simulink model "New_SPRO4"  (R2026a)
settings: Solver=FixedStepAuto  StopTime=8  RelTol=1e-6
libraries: simulink x1, slpidlib x1
settings OptimizationCC: UseDivisionForNetSlopeComputation=on  GainParamInheritBuiltInType=on  UseFloatMulNetSlope=on  InlineInvariantSignals=on  NoFixptDivByZeroProtection=on  EfficientFloat2IntCast=on  LifeSpan=1
settings RTWCC: SystemTargetFile=ert.tlc  GenerateReport=on  Toolchain=ESP32  LaunchReport=on  Description=Embedded Coder
settings CodeAppCC: CustomSymbolStrGlobalVar=rt$N$M  CustomSymbolStrType=$N$M  CustomSymbolStrFcn=$N$M$F  CustomSymbolStrMacro=$N$M
settings ERTTargetCC: ERTFilePackagingFormat=CompactWithDataFile  GenerateSampleERTMain=on  IncludeMdlTerminateFcn=off  CombineSignalStateStructs=on  SupportAbsoluteTime=off  SupportComplex=off  SupportContinuousTime=on

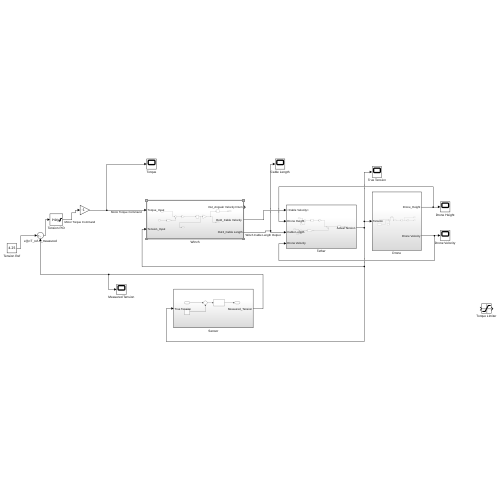
[thumbnail: Simulink's stored preview of the top-level diagram]
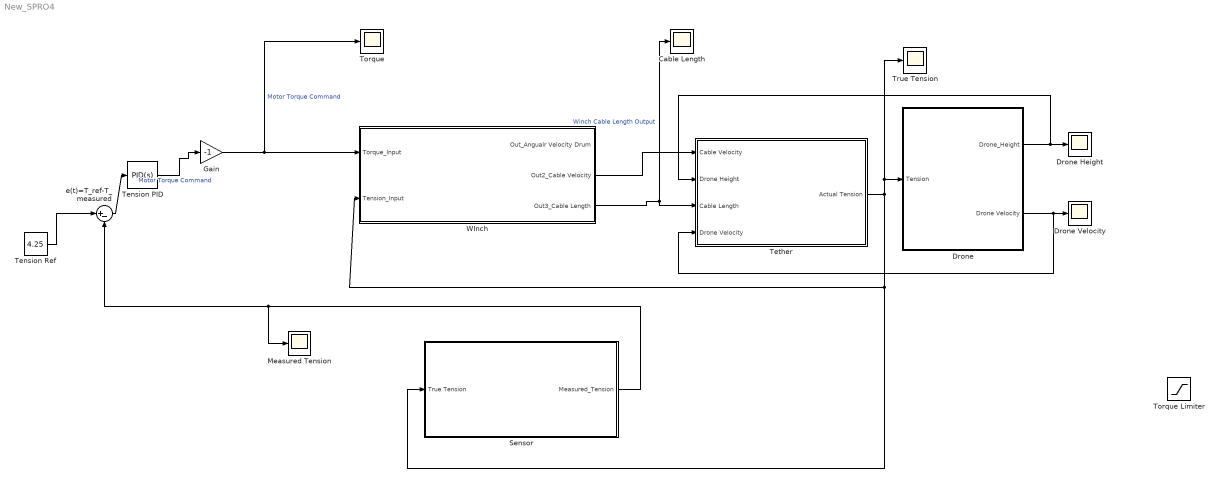
== system New_SPRO4 ==
  Cable Length : Scope
      settings: ActiveDisplayYMinimum=-13.075945732793034  ActiveDisplayYMaximum=11.241645498772957  DataLoggingVariableName=ScopeData5
  Drone : Subsystem
  Drone Height : Scope
      settings: ActiveDisplayYMinimum=-2.5970281910431563  ActiveDisplayYMaximum=9.2410311502356173  DataLoggingVariableName=ScopeData4
  Drone Velocity : Scope
      settings: ActiveDisplayYMinimum=-6.9644358509379627  ActiveDisplayYMaximum=6.4874715690258595  DataLoggingVariableName=ScopeData2
  Gain : Gain  Gain=-1
  Measured Tension : Scope
      settings: ActiveDisplayYMinimum=-21.256641439910606  ActiveDisplayYMaximum=16.681859235663254
  Sensor : Subsystem
  Tension PID : slpidlib/PID Controller  Controller=PID  Form=Parallel  TimeDomain=Continuous-time  UseExternalTs=off  SampleTime=-1  IntegratorMethod=Forward Euler  FilterMethod=Forward Euler  ControllerParametersSource=internal  P=0.005  I=0.002  UseKiTs=off  D=0.001  UseExternalDerivativeSource=off  N=10  UseFilter=on  TunerSelectOption=Transfer Function Based (PID Tuner App)  InitialConditionSource=internal  InitialConditionForIntegrator=0  InitialConditionForFilter=0  DifferentiatorICPrevScaledInput=0  ExternalReset=none  TrackingMode=off  Kt=1  LimitOutput=on  SatLimitsSource=internal  UpperSaturationLimit=0.0084  LowerSaturationLimit=-0.0084  LinearizeAsGain=on  AntiWindupMode=clamping  Kb=1  LimitIntegrator=on  UpperIntegratorSaturationLimit=0.0078  LowerIntegratorSaturationLimit=-0.0078  POutMin=[]  POutMax=[]  IOutMin=[]  IOutMax=[]  DOutMin=[]  DOutMax=[]  NOutMin=[]  NOutMax=[]  SumOutMin=[]  SumOutMax=[]  SaturationOutMin=[]  SaturationOutMax=[]  PParamMin=[]  PParamMax=[]  IParamMin=[]  IParamMax=[]  DParamMin=[]  DParamMax=[]  NParamMin=[]  NParamMax=[]  KbParamMin=[]  KbParamMax=[]  KtParamMin=[]  KtParamMax=[]  KbOutMin=[]  KbOutMax=[]  KtOutMin=[]  KtOutMax=[]  IntegratorOutMin=[]  IntegratorOutMax=[]  FilterOutMin=[]  FilterOutMax=[]  SumI1OutMin=[]  SumI1OutMax=[]  SumI2OutMin=[]  SumI2OutMax=[]  SumI3OutMin=[]  SumI3OutMax=[]  SumI4OutMin=[]  SumI4OutMax=[]  SumDOutMin=[]  SumDOutMax=[]  DifferentiatorOutMin=[]  DifferentiatorOutMax=[]  FilterDiffOutCoefMin=[]  FilterDiffOutCoefMax=[]  ReciprocalOutMin=[]  ReciprocalOutMax=[]  SumDenOutMin=[]  SumDenOutMax=[]  SumNumOutMin=[]  SumNumOutMax=[]  DivideOutMin=[]  DivideOutMax=[]  UdiffTsProdOutMin=[]  UdiffTsProdOutMax=[]  NTsProdOutMin=[]  NTsProdOutMax=[]  UintegralTsProdOutMin=[]  UintegralTsProdOutMax=[]  UngainTsProdOutMin=[]  UngainTsProdOutMax=[]  ClampingZeroOutDataTypeStr=Inherit: Inherit via back propagation  ClampingZeroOutMin=[]  ClampingZeroOutMax=[]  FilterDenConstantOutDataTypeStr=Inherit: Inherit via back propagation  FilterDenConstantOutMin=[]  FilterDenConstantOutMax=[]  PCopyOutDataTypeStr=Inherit: Inherit via back propagation  PCopyOutMin=[]  PCopyOutMax=[]  NCopyOutDataTypeStr=Inherit: Inherit via back propagation  NCopyOutMin=[]  NCopyOutMax=[]  IntegratorContinuousStateAttributes=''  IntegratorStateMustResolveToSignalObject=off  IntegratorRTWStateStorageClass=Auto  FilterContinuousStateAttributes=''  FilterStateMustResolveToSignalObject=off  FilterRTWStateStorageClass=Auto  ParallelPVariant=InternalParameters  IdealPVariant=Disabled  IVariant=InternalParameters  DVariant=InternalParameters  IntegratorVariant=Continuous  SatVariant=Enabled  AWVariant=ContClampingParallel  PCopyVariant=Disabled  TRVariant=Disabled  FdbkBlocksVariant=Forward  IdealPFdbkVariant=Disabled  SatFdbkVariant=Disabled  DerivativeFilterVariant=ContFilter  NVariant=InternalParameters  NCopyVariant=Disabled  FilterICVariant=InternalICsFilter  IntegratorICVariant=InternalICs  ExternalResetVariant=Disabled  TRSumVariant=Passthrough  SumFdbkVariant=Disabled  SumVariant=Sum_PID  TsampFilterVariant=InternalTs  TsampNgainVariant=Passthrough  TsampIntegralVariant=Disabled_SignalSpec  ExternalSaturationOutDataTypeStr=Inherit: Same as second input  DerivativeSourceVariant=ErrorSignal  PreIntVariant=InternalPreInt
  Tension Ref : Constant  Value=4.25
  Tether : Subsystem
  Torque : Scope
      settings: ActiveDisplayYMinimum=-0.022412024196520747  ActiveDisplayYMaximum=0.011746234700967979
  Torque Limiter : Saturate  UpperLimit=0.0078  LowerLimit=-0.0078
  True Tension : Scope
      settings: ActiveDisplayYMinimum=-0.060712447247646573  ActiveDisplayYMaximum=5.1920611495530729  DataLoggingVariableName=ScopeData3
  WInch : Subsystem
  e(t)=T_ref-T_measured : Sum  Inputs=|+-
  wires:
  Drone/1(Drone_Height) -> Tether/2(Drone Height), Drone Height/1
  WInch/2("Out2_Cable Velocity ") -> Tether/1("Cable Velocity ")
  Sensor/1(Measured_Tension) -> Measured Tension/1, e(t)=T_ref-T_measured/2
  WInch/3(Out3_Cable Length) -> Tether/3(Cable Length), Cable Length/1  "Winch Cable Length Output"
  Drone/2(Drone Velocity) -> Tether/4(Drone Velocity), Drone Velocity/1
  Tether/1(Actual Tension) -> True Tension/1, Drone/1(Tension), Sensor/1(True Tension), WInch/2(Tension_Input)
  e(t)=T_ref-T_measured/1 -> Tension PID/1
  Tension Ref/1 -> e(t)=T_ref-T_measured/1
  Gain/1 -> Torque/1, WInch/1(Torque_Input)  "Motor Torque Command"
  Tension PID/1 -> Gain/1  "Motor Torque Command"

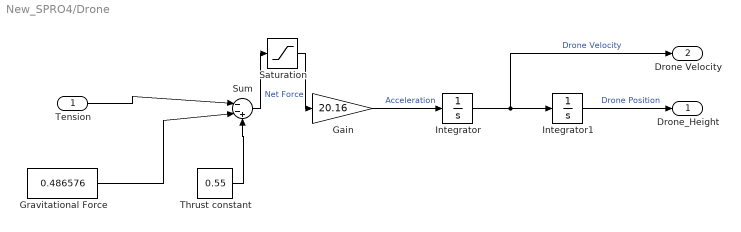
== system New_SPRO4/Drone ==
  Tension : Inport
  Gain : Gain  Gain=20.16
  Gravitational Force : Constant  Value=0.486576
  Integrator : Integrator  LimitOutput=on  UpperSaturationLimit=2  LowerSaturationLimit=-2
  Integrator1 : Integrator  InitialCondition=1.8  LimitOutput=on  UpperSaturationLimit=10  LowerSaturationLimit=0
  Saturation : Saturate  UpperLimit=5  LowerLimit=-5
  Sum : Sum  Inputs=|--+
  Thrust constant : Constant  Value=0.55
  Drone_Height : Outport
  Drone Velocity : Outport  Port=2
  wires:
  Tension/1 -> Sum/1
  Thrust constant/1 -> Sum/3
  Gravitational Force/1 -> Sum/2
  Sum/1 -> Saturation/1  "Net Force"
  Gain/1 -> Integrator/1  "Acceleration"
  Integrator/1 -> Drone Velocity/1, Integrator1/1  "Drone Velocity"
  Integrator1/1 -> Drone_Height/1  "Drone Position"
  Saturation/1 -> Gain/1

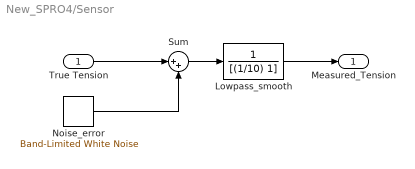
== system New_SPRO4/Sensor ==
  True Tension : Inport
  Lowpass_smooth : TransferFcn  Denominator=[(1/10) 1]
  Noise_error : simulink/Sources/Band-Limited White Noise  Cov=[0.0000004318]  Ts=0.1  seed=[23341]
  Sum : Sum  Inputs=|++
  Measured_Tension : Outport
  wires:
  True Tension/1 -> Sum/1
  Noise_error/1 -> Sum/2
  Sum/1 -> Lowpass_smooth/1
  Lowpass_smooth/1 -> Measured_Tension/1

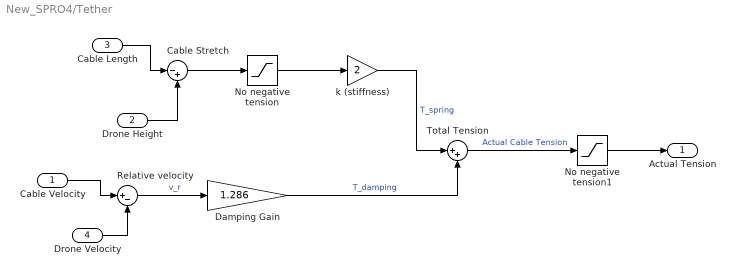
== system New_SPRO4/Tether ==
  "Cable Velocity " : Inport
  Drone Height : Inport  Port=2
  Cable Length : Inport  Port=3
  Drone Velocity : Inport  Port=4
  Cable Stretch : Sum  Inputs=|-+
  Damping Gain : Gain  Gain=1.286
  No negative tension : Saturate  UpperLimit=inf  LowerLimit=0
  No negative tension1 : Saturate  UpperLimit=inf  LowerLimit=0
  Relative velocity : Sum  Inputs=|+-
  Total Tension : Sum  Inputs=|++
  k (stiffness) : Gain  Gain=2
  Actual Tension : Outport
  wires:
  Drone Height/1 -> Cable Stretch/2
  Cable Length/1 -> Cable Stretch/1
  Cable Stretch/1 -> No negative tension/1
  No negative tension/1 -> k (stiffness)/1
  Drone Velocity/1 -> Relative velocity/2
  Relative velocity/1 -> Damping Gain/1  "v_r"
  k (stiffness)/1 -> Total Tension/1  "T_spring"
  Damping Gain/1 -> Total Tension/2  "T_damping"
  Total Tension/1 -> No negative tension1/1  "Actual Cable Tension"
  No negative tension1/1 -> Actual Tension/1
  "Cable Velocity "/1 -> Relative velocity/1

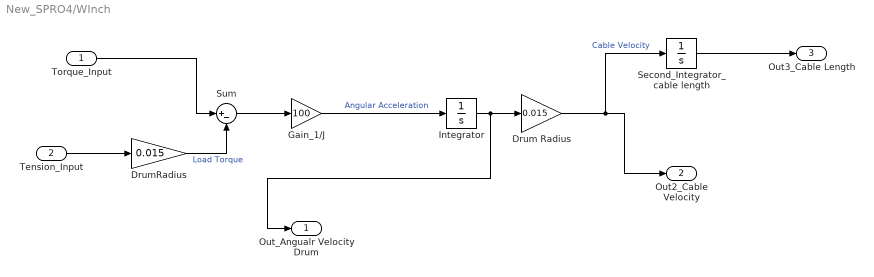
== system New_SPRO4/WInch ==
  Torque_Input : Inport
  Tension_Input : Inport  Port=2
  Drum Radius : Gain  Gain=0.015
  DrumRadius : Gain  Gain=0.015
  Gain_1/J : Gain  Gain=100
  Integrator : Integrator
  Second_Integrator_cable length : Integrator  InitialCondition=1.8
  Sum : Sum  Inputs=|+-
  Out_Angualr Velocity Drum : Outport
  "Out2_Cable Velocity " : Outport  Port=2
  Out3_Cable Length : Outport  Port=3
  wires:
  Gain_1/J/1 -> Integrator/1  "Angular Acceleration"
  Integrator/1 -> Drum Radius/1, Out_Angualr Velocity Drum/1
  Drum Radius/1 -> Second_Integrator_cable length/1, "Out2_Cable Velocity "/1  "Cable Velocity"
  Second_Integrator_cable length/1 -> Out3_Cable Length/1
  Tension_Input/1 -> DrumRadius/1
  DrumRadius/1 -> Sum/2  "Load Torque"
  Sum/1 -> Gain_1/J/1
  Torque_Input/1 -> Sum/1
